simulink model "cntrl_sim"  (R2021a)
settings: Solver=ode23tb  StartTime=0.0  StopTime=Tsim  MaxStep=1e-3  RelTol=1e-3
values from neighbouring files (symbols this model uses):
  Dw = 5e-3*[1 1 1].'    [cntrl_ini.m]
  Jinv = diag(1./J)    [cntrl_ini.m]
  k = [krp krp ky]    [cntrl_ini.m]
  Kp = [1 1 1]*0.9    [cntrl_ini.m]
  quat_0 = rpy2quat(rpy_0)    [cntrl_ini.m]
  rpy_setp = [75, 65, 0] * pi/180    [cntrl_ini.m]
  Tsave = Tsim / 50    (= 0.003)    [cntrl_ini.m]
libraries: cstblocks x24
settings Model: Creator=pmic  LastModifiedBy=pmic
settings DataIOCC: ReturnWorkspaceOutputs=off

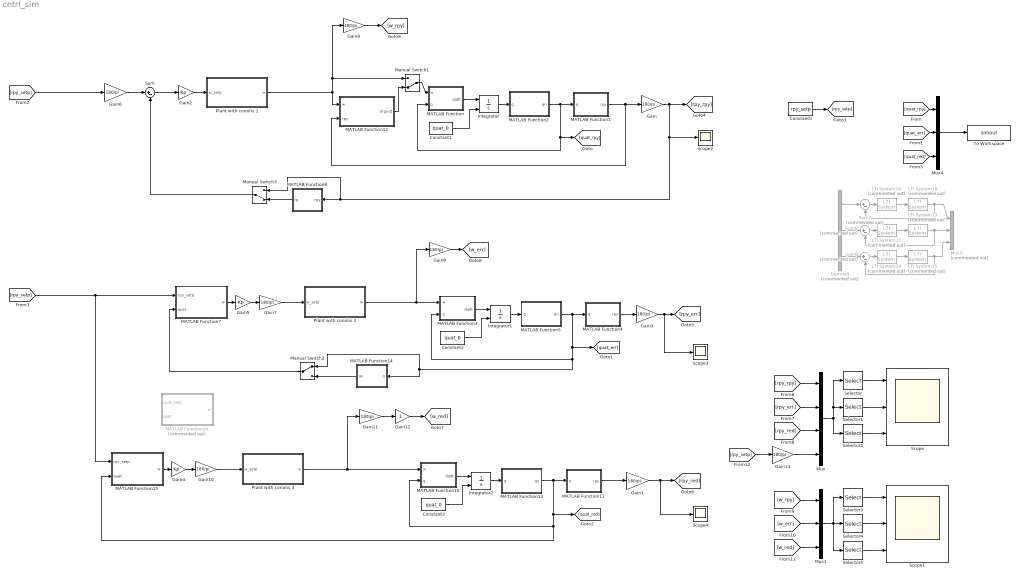
== system cntrl_sim ==
  Constant1 : Constant  Value=quat_0
  Constant2 : Constant  Value=quat_0
  Constant3 : Constant  Value=quat_0
  Constant5 : Constant  Value=rpy_setp
  Demux8 : Demux  Commented=on  Outputs=3
  Gain{,1,3,6..11,14} (10 alike) : Gain  Gain=180/pi
  Gain12 : Gain
  Gain2 : Gain  Gain=Kp
  Gain4 : Gain  Gain=Kp
  Gain5 : Gain  Gain=Kp
  Integrator : Integrator  InitialConditionSource=external  InitialCondition=[1 0 0 0]
  Integrator1 : Integrator  InitialConditionSource=external  InitialCondition=[1 0 0 0]
  Integrator2 : Integrator  InitialConditionSource=external  InitialCondition=[1 0 0 0]
  LTI System13 : cstblocks/LTI System  Commented=on  sys=Prp  IC=[]
  LTI System14 : cstblocks/LTI System  Commented=on  sys=Cy  IC=[]
  LTI System15 : cstblocks/LTI System  Commented=on  sys=Py  IC=[]
  LTI System16 : cstblocks/LTI System  Commented=on  sys=Crp  IC=[]
  LTI System17 : cstblocks/LTI System  Commented=on  sys=Crp  IC=[]
  LTI System18 : cstblocks/LTI System  Commented=on  sys=Prp  IC=[]
  MATLAB Function : MATLAB Function  TreatAsAtomicUnit=on
  MATLAB Function1 : MATLAB Function  TreatAsAtomicUnit=on
  MATLAB Function10 : MATLAB Function  TreatAsAtomicUnit=on
  MATLAB Function11 : MATLAB Function  TreatAsAtomicUnit=on
  MATLAB Function12 : MATLAB Function  TreatAsAtomicUnit=on
  MATLAB Function13 : MATLAB Function  TreatAsAtomicUnit=on
  MATLAB Function14 : MATLAB Function  TreatAsAtomicUnit=on
  MATLAB Function15 : MATLAB Function  TreatAsAtomicUnit=on
  MATLAB Function16 : MATLAB Function  Commented=on  TreatAsAtomicUnit=on
  MATLAB Function2 : MATLAB Function  TreatAsAtomicUnit=on
  MATLAB Function3 : MATLAB Function  TreatAsAtomicUnit=on
  MATLAB Function4 : MATLAB Function  TreatAsAtomicUnit=on
  MATLAB Function5 : MATLAB Function  TreatAsAtomicUnit=on
  MATLAB Function7 : MATLAB Function  TreatAsAtomicUnit=on
  MATLAB Function8 : MATLAB Function  TreatAsAtomicUnit=on
  Manual Switch1 : ManualSwitch  CurrentSetting=0
  Manual Switch2 : ManualSwitch
  Manual Switch3 : ManualSwitch  CurrentSetting=0
  Mux : Mux
  Mux1 : Mux  Inputs=3
  Mux3 : Mux  Commented=on  Inputs=3
  Mux4 : Mux  Inputs=3
  Plant with coriolis 1 : Subsystem
  Plant with coriolis 2 : Subsystem
  Plant with coriolis 3 : Subsystem
  Scope : Scope  NumInputPorts=3
  Scope1 : Scope  NumInputPorts=3
  Scope2 : Scope
  Scope3 : Scope
  Scope4 : Scope
  Selector : Selector  InputPortWidth=12  IndexOptions=Index vector (dialog)  Indices=[1 4 7 10]+0  OutputSizes=1
  Selector1 : Selector  InputPortWidth=12  IndexOptions=Index vector (dialog)  Indices=[1 4 7 10]+1  OutputSizes=1
  Selector2 : Selector  InputPortWidth=12  IndexOptions=Index vector (dialog)  Indices=[1 4 7 10]+2  OutputSizes=1
  Selector3 : Selector  InputPortWidth=9  IndexOptions=Index vector (dialog)  Indices=[1 4 7]+0  OutputSizes=1
  Selector4 : Selector  InputPortWidth=9  IndexOptions=Index vector (dialog)  Indices=[1 4 7]+1  OutputSizes=1
  Selector5 : Selector  InputPortWidth=9  IndexOptions=Index vector (dialog)  Indices=[1 4 7]+2  OutputSizes=1
  Sum : Sum  Inputs=|+-
  Sum7 : Sum  Commented=on  Inputs=|+-
  Sum8 : Sum  Commented=on  Inputs=|+-
  Sum9 : Sum  Commented=on  Inputs=|+-
  To Workspace : ToWorkspace  VariableName=simout  SaveFormat=Structure With Time  SampleTime=Tsave
  wires:
  Constant1/1 -> Integrator/2
  MATLAB Function/1(dqdt) -> Integrator/1
  Integrator/1 -> MATLAB Function2/1(q)
  MATLAB Function1/1(rpy) -> MATLAB Function12/2(rpy), Gain/1
  Sum/1 -> Gain2/1
  MATLAB Function4/1(rpy) -> Gain3/1
  Gain5/1 -> Gain7/1
  MATLAB Function7/1(w) -> Gain5/1
  Mux4/1 -> To Workspace/1
  MATLAB Function2/1(qn) -> MATLAB Function1/1(q), MATLAB Function/2(q), [quat_rpy]
  Plant with coriolis 2/1(w) -> MATLAB Function3/1(w), Gain9/1
  Plant with coriolis 1/1(w) -> MATLAB Function12/1(w), Manual Switch1/1, Gain8/1
  Manual Switch1/1 -> MATLAB Function/1(w)
  MATLAB Function12/1(drpydt) -> Manual Switch1/2
  Gain6/1 -> Sum/1
  LTI System17/1 -> LTI System13/1
  LTI System13/1 -> Sum8/2, Mux3/2
  Demux8/3 -> Sum9/1
  LTI System15/1 -> Sum9/2, Mux3/3
  Sum8/1 -> LTI System17/1
  LTI System16/1 -> LTI System18/1
  LTI System14/1 -> LTI System15/1
  Demux8/2 -> Sum8/1
  Sum9/1 -> LTI System14/1
  Sum7/1 -> LTI System16/1
  LTI System18/1 -> Mux3/1, Sum7/2
  Demux8/1 -> Sum7/1
  Gain2/1 -> Plant with coriolis 1/1(w_setp)
  Gain7/1 -> Plant with coriolis 2/1(w_setp)
  [quat_rpy] -> Mux4/1
  MATLAB Function5/1(qn) -> MATLAB Function4/1(q), [quat_err], Manual Switch2/1, MATLAB Function14/1(q), MATLAB Function3/2(q)
  MATLAB Function3/1(dqdt) -> Integrator1/1
  Integrator1/1 -> MATLAB Function5/1(q)
  Constant2/1 -> Integrator1/2
  [quat_err] -> Mux4/2
  Constant3/1 -> Integrator2/2
  Integrator2/1 -> MATLAB Function13/1(q)
  MATLAB Function10/1(dqdt) -> Integrator2/1
  Gain10/1 -> Plant with coriolis 3/1(w_setp)
  Plant with coriolis 3/1(w) -> Gain11/1, MATLAB Function10/1(w)
  MATLAB Function13/1(qn) -> MATLAB Function15/2(quat), MATLAB Function10/2(q), [quat_red], MATLAB Function11/1(q)
  MATLAB Function15/1(w) -> Gain4/1
  Gain4/1 -> Gain10/1
  [rpy_setp] -> MATLAB Function15/1(rpy_setp), MATLAB Function7/1(rpy_setp)
  MATLAB Function11/1(rpy) -> Gain1/1
  Constant5/1 -> [rpy_setp]
  [rpy_setp] -> Gain6/1
  [quat_red] -> Mux4/3
  Manual Switch2/1 -> MATLAB Function7/2(quat)
  Gain3/1 -> Scope3/1, [rpy_err]
  [rpy_rpy] -> Mux/1
  [rpy_err] -> Mux/2
  [rpy_red] -> Mux/3
  Mux/1 -> Selector2/1, Selector1/1, Selector/1
  Selector/1 -> Scope/1
  Selector1/1 -> Scope/2
  Selector2/1 -> Scope/3
  Gain9/1 -> [w_err]
  Gain8/1 -> [w_rpy]
  Selector5/1 -> Scope1/3
  Selector4/1 -> Scope1/2
  Selector3/1 -> Scope1/1
  Mux1/1 -> Selector3/1, Selector4/1, Selector5/1
  [w_red] -> Mux1/3
  [w_err] -> Mux1/2
  [w_rpy] -> Mux1/1
  Gain12/1 -> [w_red]
  Gain11/1 -> Gain12/1
  Gain1/1 -> Scope4/1, [rpy_red]
  MATLAB Function8/1(rp) -> Manual Switch3/2
  Gain/1 -> [rpy_rpy], Scope2/1, Manual Switch3/1, MATLAB Function8/1(rpy)
  Manual Switch3/1 -> Sum/2
  [rpy_setp] -> Gain14/1
  Gain14/1 -> Mux/4
  MATLAB Function14/1(qn) -> Manual Switch2/2

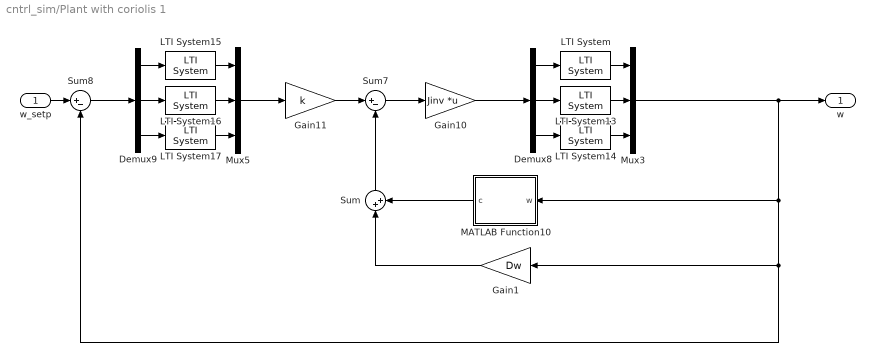
== system cntrl_sim/Plant with coriolis 1 ==
  w_setp : Inport
  Demux8 : Demux  Outputs=3
  Demux9 : Demux  Outputs=3
  Gain1 : Gain  Gain=Dw
  Gain10 : Gain  Gain=Jinv  Multiplication=Matrix(K*u)
  Gain11 : Gain  Gain=k
  LTI System : cstblocks/LTI System  sys=Prp_  IC=[]
  LTI System13 : cstblocks/LTI System  sys=Prp_  IC=[]
  LTI System14 : cstblocks/LTI System  sys=Py_  IC=[]
  LTI System15 : cstblocks/LTI System  sys=Crp  IC=[]
  LTI System16 : cstblocks/LTI System  sys=Crp  IC=[]
  LTI System17 : cstblocks/LTI System  sys=Cy  IC=[]
  MATLAB Function10 : MATLAB Function  TreatAsAtomicUnit=on
  Mux3 : Mux  Inputs=3
  Mux5 : Mux  Inputs=3
  Sum : Sum  Inputs=|++
  Sum7 : Sum  Inputs=|+-
  Sum8 : Sum  Inputs=|+-
  w : Outport
  wires:
  w_setp/1 -> Sum8/1
  Demux8/1 -> LTI System/1
  Gain10/1 -> Demux8/1
  Sum7/1 -> Gain10/1
  LTI System/1 -> Mux3/1
  LTI System14/1 -> Mux3/3
  Demux9/3 -> LTI System17/1
  Mux3/1 -> Gain1/1, Sum8/2, MATLAB Function10/1(w), w/1
  Demux9/1 -> LTI System15/1
  Gain11/1 -> Sum7/1
  LTI System17/1 -> Mux5/3
  LTI System13/1 -> Mux3/2
  Mux5/1 -> Gain11/1
  LTI System16/1 -> Mux5/2
  Sum8/1 -> Demux9/1
  Demux8/2 -> LTI System13/1
  Demux8/3 -> LTI System14/1
  Demux9/2 -> LTI System16/1
  LTI System15/1 -> Mux5/1
  Gain1/1 -> Sum/1
  MATLAB Function10/1(c) -> Sum/2
  Sum/1 -> Sum7/2

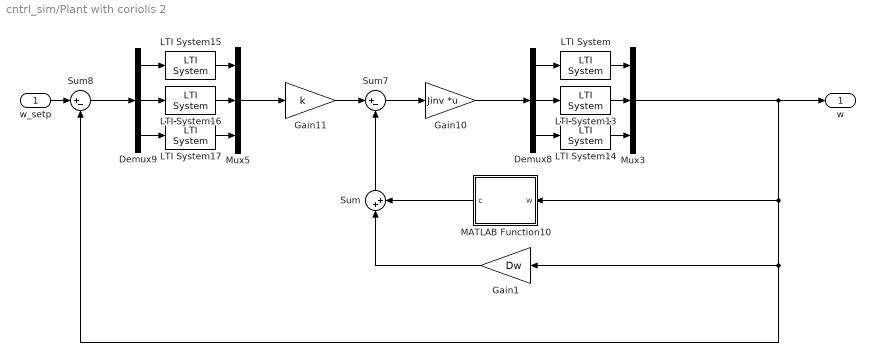
== system cntrl_sim/Plant with coriolis 2 ==
  w_setp : Inport
  Demux8 : Demux  Outputs=3
  Demux9 : Demux  Outputs=3
  Gain1 : Gain  Gain=Dw
  Gain10 : Gain  Gain=Jinv  Multiplication=Matrix(K*u)
  Gain11 : Gain  Gain=k
  LTI System : cstblocks/LTI System  sys=Prp_  IC=[]
  LTI System13 : cstblocks/LTI System  sys=Prp_  IC=[]
  LTI System14 : cstblocks/LTI System  sys=Py_  IC=[]
  LTI System15 : cstblocks/LTI System  sys=Crp  IC=[]
  LTI System16 : cstblocks/LTI System  sys=Crp  IC=[]
  LTI System17 : cstblocks/LTI System  sys=Cy  IC=[]
  MATLAB Function10 : MATLAB Function  TreatAsAtomicUnit=on
  Mux3 : Mux  Inputs=3
  Mux5 : Mux  Inputs=3
  Sum : Sum  Inputs=|++
  Sum7 : Sum  Inputs=|+-
  Sum8 : Sum  Inputs=|+-
  w : Outport
  wires:
  Sum/1 -> Sum7/2
  MATLAB Function10/1(c) -> Sum/2
  Gain1/1 -> Sum/1
  LTI System15/1 -> Mux5/1
  Demux9/2 -> LTI System16/1
  Demux8/3 -> LTI System14/1
  Demux8/2 -> LTI System13/1
  Sum8/1 -> Demux9/1
  LTI System16/1 -> Mux5/2
  Mux5/1 -> Gain11/1
  LTI System13/1 -> Mux3/2
  LTI System17/1 -> Mux5/3
  Gain11/1 -> Sum7/1
  Demux9/1 -> LTI System15/1
  Mux3/1 -> w/1, MATLAB Function10/1(w), Sum8/2, Gain1/1
  Demux9/3 -> LTI System17/1
  LTI System14/1 -> Mux3/3
  LTI System/1 -> Mux3/1
  Sum7/1 -> Gain10/1
  Gain10/1 -> Demux8/1
  Demux8/1 -> LTI System/1
  w_setp/1 -> Sum8/1

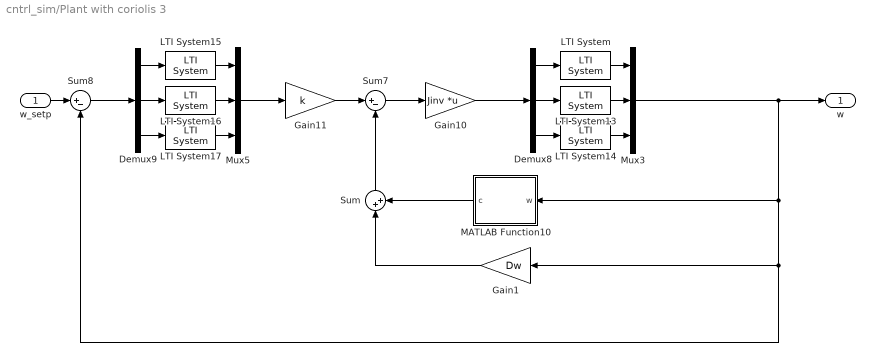
== system cntrl_sim/Plant with coriolis 3 ==
  w_setp : Inport
  Demux8 : Demux  Outputs=3
  Demux9 : Demux  Outputs=3
  Gain1 : Gain  Gain=Dw
  Gain10 : Gain  Gain=Jinv  Multiplication=Matrix(K*u)
  Gain11 : Gain  Gain=k
  LTI System : cstblocks/LTI System  sys=Prp_  IC=[]
  LTI System13 : cstblocks/LTI System  sys=Prp_  IC=[]
  LTI System14 : cstblocks/LTI System  sys=Py_  IC=[]
  LTI System15 : cstblocks/LTI System  sys=Crp  IC=[]
  LTI System16 : cstblocks/LTI System  sys=Crp  IC=[]
  LTI System17 : cstblocks/LTI System  sys=Cy  IC=[]
  MATLAB Function10 : MATLAB Function  TreatAsAtomicUnit=on
  Mux3 : Mux  Inputs=3
  Mux5 : Mux  Inputs=3
  Sum : Sum  Inputs=|++
  Sum7 : Sum  Inputs=|+-
  Sum8 : Sum  Inputs=|+-
  w : Outport
  wires:
  w_setp/1 -> Sum8/1
  Demux8/1 -> LTI System/1
  Gain10/1 -> Demux8/1
  Sum7/1 -> Gain10/1
  LTI System/1 -> Mux3/1
  LTI System14/1 -> Mux3/3
  Demux9/3 -> LTI System17/1
  Mux3/1 -> Gain1/1, Sum8/2, MATLAB Function10/1(w), w/1
  Demux9/1 -> LTI System15/1
  Gain11/1 -> Sum7/1
  LTI System17/1 -> Mux5/3
  LTI System13/1 -> Mux3/2
  Mux5/1 -> Gain11/1
  LTI System16/1 -> Mux5/2
  Sum8/1 -> Demux9/1
  Demux8/2 -> LTI System13/1
  Demux8/3 -> LTI System14/1
  Demux9/2 -> LTI System16/1
  LTI System15/1 -> Mux5/1
  Gain1/1 -> Sum/1
  MATLAB Function10/1(c) -> Sum/2
  Sum/1 -> Sum7/2

== matlab function cntrl_sim/Plant with coriolis 1/MATLAB Function10 ==
  data: w input; c output; J parameter
function c = coriolis(w, J)

c = cross( w, J .* w );

end

== matlab function cntrl_sim/MATLAB Function13 ==
  data: q input; qn output
function qn = quat_normalise(q)

qn = q;
n = norm(qn);
if n > 0
    qn = qn ./ n;
end

end

== matlab function cntrl_sim/MATLAB Function14 ==
  data: q input; qn output
function qn = remove_yaw(q)

% CEB = quat2CEB(q);
% psi = quat2psi(q);
% Cz = [[cos(psi) -sin(psi) 0]; [sin(psi) cos(psi) 0]; [0 0 1]];
% q = rotm2quat(Cz' * CEB);

psi = quat2psi(q);
qz = [cos(psi/2); 0; 0; -sin(psi/2)];
q = ( quat2QprodL(qz) * q );

qn = q;
n = norm(qn);
if n > 0
    qn = qn ./ n;
end

end

function psi = quat2psi(q)

    psi  = atan2( (q(2).*q(3) + q(1).*q(4) ), 0.5 - (q(3).^2 + q(4).^2) );
    % pai = atan2( 2*(q(2).*q(3)+q(1).*q(4)), q(1).^2 + q(2).^2 - q(3).^2 - q(4).^2 );
    
end

== matlab function cntrl_sim/MATLAB Function15 ==
  data: rpy_setp input; w output; quat input
function w = quatError2w(rpy_setp, quat)

% extract only rp from rpy setp
r = rpy_setp(1); % - those are available in pid.c
p = rpy_setp(2);

% rotate ez into body frame
% CEB = [cos(psi)*cos(theta), cos(psi)*sin(phi)*sin(theta) - cos(phi)*sin(psi), sin(phi)*sin(psi) + cos(phi)*cos(psi)*sin(theta)]
%       [cos(theta)*sin(psi), cos(phi)*cos(psi) + sin(phi)*sin(psi)*sin(theta), cos(phi)*sin(psi)*sin(theta) - cos(psi)*sin(phi)]
%       [        -sin(theta),                              cos(theta)*sin(phi),                              cos(phi)*cos(theta)]
sr = sin(r); sp = sin(p);
cr = cos(r); cp = cos(p);
CEB = quat2CEB(quat); % - this is available in imu.c
ez_des = CEB.' * [ cr*sp; -sr; cr*cp];

% calculate angle and rotation vector
ang = acos(ez_des(3));
v = [-ez_des(2); ez_des(1)];
v_norm_squared = ez_des(1)^2 + ez_des(2)^2;

if abs(ang) > 1e-6
    ax = v;
    if v_norm_squared >= 1e-6
        ax = ax ./ sqrt(v_norm_squared);
    end
    w = ang * [ax; 0];
else
    w = [0; 0; 0];
end

end

== matlab function cntrl_sim/MATLAB Function16 ==
  data: quat_setp input; w output; quat input
function w = quatError2w(quat_setp, quat)

CEB_setp = quat2CEB(quat_setp);
CEB      = quat2CEB(quat);

psi_setp = quat2psi(quat_setp);
psi      = quat2psi(quat);
Cz_setp = [[cos(psi_setp) -sin(psi_setp) 0]; [sin(psi_setp) cos(psi_setp) 0]; [0 0 1]];
Cz      = [[cos(psi) -sin(psi) 0]; [sin(psi) cos(psi) 0]; [0 0 1]];

% % CEB_setp = Cz_setp.' * CEB_setp;
% % quat_setp = rotm2quat(CEB_setp);
% CEB = Cz.' * CEB;
% quat = rotm2quat(CEB);

CEB_setp = Cz.' * CEB_setp;
quat_setp = rotm2quat(CEB_setp);

% CEB = Cz_setp.' * CEB;
% quat = rotm2quat(CEB);

quat_conj = quat; quat_conj(2:4) = -quat_conj(2:4);
quat_error = ( quat2QprodL(quat_conj) * quat_setp.' ).';
ang = 2 * atan2( norm( quat_error(2:4) ), quat_error(1) );
ax = [1 0 0];
if abs(ang) > 1e-6
    ax = quat_error(2:4) / sin( ang / 2 );
end
w = ang * ax;

end

function psi = quat2psi(q)

    psi = atan2( (q(2).*q(3) + q(1).*q(4) ), 0.5 - (q(3).^2 + q(4).^2) );

end

== matlab function cntrl_sim/MATLAB Function ==
  data: w input; dqdt output; q input
function dqdt = calc_dqdt(w, q)

dqdt = 0.5 * quat2QprodL(q) * [0; w];

end

== matlab function cntrl_sim/MATLAB Function2 ==
  data: q input; qn output
function qn = quat_normalise(q)

qn = q;
n = norm(qn);
if n > 0
    qn = qn ./ n;
end

end

== matlab function cntrl_sim/MATLAB Function3 ==
  data: w input; dqdt output; q input
function dqdt = calc_dqdt(w, q)

dqdt = 0.5 * quat2QprodL(q) * [0; w];

end

== matlab function cntrl_sim/MATLAB Function4 ==
  data: q input; rpy output
function rpy = quat2rpy(q)

rpy = [quat2phi(q); quat2theta(q); quat2psi(q)];
% rpy = atan2( sin(rpy), cos(rpy) );

end

function phi = quat2phi(q)

    phi = atan2( (q(3).*q(4) + q(1).*q(2) ), 0.5 - (q(2).^2 + q(3).^2) );
    
end

function theta = quat2theta(q)

    sinarg = -2*(q(2).*q(4) - q(1).*q(3));
    sinarg(sinarg > 1) = 1;
    sinarg(sinarg < -1) = -1;
    theta = asin(sinarg);

end

function psi = quat2psi(q)

    psi = atan2( (q(2).*q(3) + q(1).*q(4) ), 0.5 - (q(3).^2 + q(4).^2) );

end

== matlab function cntrl_sim/MATLAB Function5 ==
  data: q input; qn output
function qn = quat_normalise(q)

qn = q;
n = norm(qn);
if n > 0
    qn = qn ./ n;
end

end

== matlab function cntrl_sim/Plant with coriolis 2/MATLAB Function10 ==
  data: w input; c output; J parameter
function c = coriolis(w, J)

c = cross( w, J .* w );

end

== matlab function cntrl_sim/MATLAB Function7 ==
  data: rpy_setp input; w output; quat input
function w = quatError2w(rpy_setp, quat)

quat_setp = rpy2quat(rpy_setp);

quat_conj = quat; quat_conj(2:4) = -quat_conj(2:4);
quat_error = ( quat2QprodL(quat_conj) * quat_setp );
ang = 2 * atan2( norm( quat_error(2:4) ), quat_error(1) );
if abs(ang) > 1e-6
    w = ang * quat_error(2:4) ./ sin( ang / 2 );
else
    w = [0; 0; 1];
end

end

function q = rpy2quat(rpy)

    c = cos(rpy/2);
    s = sin(rpy/2);
    q = [c(3)*c(2)*c(1) + s(3)*s(2)*s(1); ...
         c(3)*c(2)*s(1) - s(3)*s(2)*c(1); ...
         c(3)*s(2)*c(1) + s(3)*c(2)*s(1); ...
         s(3)*c(2)*c(1) - c(3)*s(2)*s(1)];

end

== matlab function cntrl_sim/MATLAB Function8 ==
  data: rpy input; rp output
function rp = remove_yaw(rpy)

rp = rpy;
rp(3) = 0;

end

== matlab function cntrl_sim/Plant with coriolis 3/MATLAB Function10 ==
  data: w input; c output; J parameter
function c = coriolis(w, J)

c = cross( w, J .* w );

end

== matlab function cntrl_sim/MATLAB Function1 ==
  data: q input; rpy output
function rpy = quat2rpy(q)

rpy = [quat2phi(q); quat2theta(q); quat2psi(q)];
% rpy = atan2( sin(rpy), cos(rpy) );

end

function phi = quat2phi(q)

    phi = atan2( (q(3).*q(4) + q(1).*q(2) ), 0.5 - (q(2).^2 + q(3).^2) );
    
end

function theta = quat2theta(q)

    sinarg = -2*(q(2).*q(4) - q(1).*q(3));
    sinarg(sinarg > 1) = 1;
    sinarg(sinarg < -1) = -1;
    theta = asin(sinarg);

end

function psi = quat2psi(q)

    psi = atan2( (q(2).*q(3) + q(1).*q(4) ), 0.5 - (q(3).^2 + q(4).^2) );

end

== matlab function cntrl_sim/MATLAB Function10 ==
  data: w input; dqdt output; q input
function dqdt = calc_dqdt(w, q)

dqdt = 0.5 * quat2QprodL(q) * [0; w];

end

== matlab function cntrl_sim/MATLAB Function11 ==
  data: q input; rpy output
function rpy = quat2rpy(q)

rpy = [quat2phi(q); quat2theta(q); quat2psi(q)];
% rpy = atan2( sin(rpy), cos(rpy) );

end

function phi = quat2phi(q)

    phi = atan2( (q(3).*q(4) + q(1).*q(2) ), 0.5 - (q(2).^2 + q(3).^2) );
    
end

function theta = quat2theta(q)

    sinarg = -2*(q(2).*q(4) - q(1).*q(3));
    sinarg(sinarg > 1) = 1;
    sinarg(sinarg < -1) = -1;
    theta = asin(sinarg);

end

function psi = quat2psi(q)

    psi = atan2( (q(2).*q(3) + q(1).*q(4) ), 0.5 - (q(3).^2 + q(4).^2) );

end

== matlab function cntrl_sim/MATLAB Function12 ==
  data: w input; drpydt output; rpy input
function drpydt = calc_drpydt_inv(w, rpy)

phi   = rpy(1);
theta = rpy(2);
psi   = rpy(3);

% jacobian earth to body angle velocities
JBE = [[1,         0,         -sin(theta)]; ...
       [0,  cos(phi), cos(theta)*sin(phi)]; ...
       [0, -sin(phi), cos(theta)*cos(phi)]];

drpydt = JBE * w;
   
end
